simulink model "BATTERYLESS_SOLAR_INVERTER_DRIVE"  (R2021a)
settings: Solver=ode15s  StartTime=0.0  StopTime=inf  FixedStep=.00001  MaxStep=.00001  RelTol=1e-3  EnableMultiTasking=on
undefined symbols (not defined in the file): Capacitor, dEgdT, EgRef, gcbh, k1, Rsh_array5pc, Run, sps_rtmsupport, Start, Tref_K, VT_ref
libraries: fl_lib x7, spsCurrentMeasurementLib x6, nesl_utility x6, sh_lib x5, spsSeriesRLCBranchLib x5, spsIGBTDiodeLib x4, spsVoltageMeasurementLib x4, pid_lib x3, spsPVarrayModel x3, simulink x3, spsControlledCurrentSourceLib x2, spsRMSLib x2
(part 5 of 5)

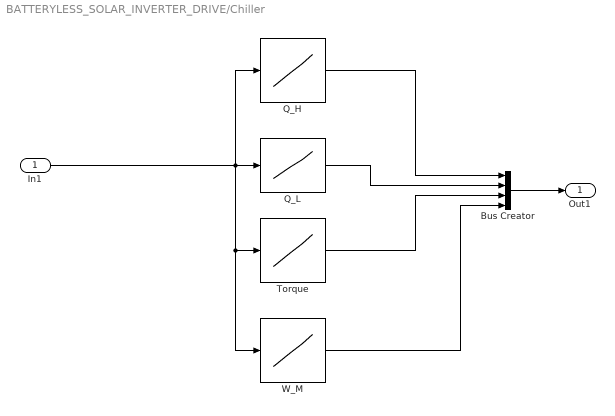
== system BATTERYLESS_SOLAR_INVERTER_DRIVE/Chiller ==
  In1 : Inport
  Bus Creator : BusCreator  Inputs=4
  Q_H : Lookup_n-D  NumberOfTableDimensions=1  BreakpointsForDimension1=|  Table=|  InternalRulePriority=Speed  RndMeth=Simplest  InputSameDT=on
      BreakpointsForDimension1=|
      | [0.16
      | 2.16
      | 4.16
      | 6.16
      | 8.16
      | 10.16
      | 12.16
      | 14.16
      | 16.16
      | 18.16
      | 20.16
      | 22.16
      | 24.16
      | 26.16
      | 28.16
      | 30.16
      | 32.16
      | 34.16
      | 36.16
      | 38.16
      | 40.16
      | 42.16
      | 44.16
      | 46.16
      | 48.16
      | 50.16
      | 52.16
      | 54.16
      | 56.16
      | 58.16
      | 60.16
      | 62.16
      | 64.16
      | 66.16
      | 68.16
      | 70.16
      | 72.16
      | 74.16
      | 76.16
      | 78.16
      | 80.16
      | 82.16
      | 84.16
      | 86.16
      | 88.16
      | 90.16
      | 92.16
      | 94.16
      | 96.16
      | 98.16
      | 100.2
      | 102.2
      | 104.2
      | 106.2
      | 108.2
      | 110.2
      | 112.2
      | 114.2
      | 116.2
      | 118.2
      | 120.2
      | 122.2
      | 124.2
      | 126.2
      | 128.2
      | 130.2
      | 132.2
      | 134.2
      | 136.2
      | 138.2
      | 140.2
      | 142.2
      | 144.2
      | 146.2
      | 148.2
      | 150.2
      | 152.2
      | 154.2
      | 156.2
      | 158.2
      | 160.2
      | 162.2
      | 164.2
      | 166.2
      | 168.2
      | 170.2
      | 172.2
      | 174.2
      | 176.2
      | 178.2
      | 180.2
      | 182.2
      | 184.2
      | 186.2
      | 188.2
      | 190.2
      | 192.2
      | 194.2
      | 196.2
      | 198.2
      | 200.2
      | 202.2
      | 204.2
      | 206.2
      | 208.2
      | 210.2
      | 212.2
      | 214.2
      | 216.2
      | 218.2
      | 220.2
      | 222.2
      | 224.2
      | 226.2
      | 228.2
      | 230.2
      | 232.2
      | 234.2
      | 236.2
      | 238.2
      | 240.2
      | 242.2
      | 244.2
      | 246.2
      | 248.2
      | 250.2
      | 252.2
      | 254.2
      | 256.2
      | 258.2
      | 260.2
      | 262.2
      | 264.2
      | 266.2
      | 268.2
      | 270.2
      | 272.2
      | 274.2
      | 276.2
      | 278.2
      | 280.2
      | 282.2
      | 284.2
      | 286.2
      | 288.2
      | 290.2
      | 292.2
      | 294.2
      | 296.2
      | 298.2
      | 300.2
      | 302.2
      | 304.2
      | 306.2
      | 308.2
      | 310.2
      | 312.2
      | 314.2
      | ]
      Table=|
      | [0.6508
      | 8.784
      | 16.92
      | 25.05
      | 33.18
      | 41.31
      | 49.43
      | 57.55
      | 65.67
      | 73.78
      | 81.88
      | 89.98
      | 98.07
      | 106.2
      | 114.2
      | 122.3
      | 130.4
      | 138.4
      | 146.4
      | 154.5
      | 162.5
      | 170.5
      | 178.5
      | 186.4
      | 194.4
      | 202.4
      | 210.3
      | 218.2
      | 226.1
      | 234
      | 241.9
      | 249.7
      | 257.6
      | 265.4
      | 273.2
      | 281
      | 288.8
      | 296.5
      | 304.2
      | 312
      | 319.6
      | 327.3
      | 335
      | 342.6
      | 350.2
      | 357.8
      | 365.4
      | 372.9
      | 380.4
      | 387.9
      | 395.4
      | 402.8
      | 410.3
      | 417.7
      | 425.1
      | 432.4
      | 439.8
      | 447.1
      | 454.4
      | 461.6
      | 468.9
      | 476.1
      | 483.3
      | 490.4
      | 497.6
      | 504.7
      | 511.8
      | 518.8
      | 525.9
      | 532.9
      | 539.9
      | 546.8
      | 553.8
      | 560.7
      | 567.5
      | 574.4
      | 581.2
      | 588
      | 594.8
      | 601.5
      | 608.2
      | 614.9
      | 621.6
      | 628.2
      | 634.8
      | 641.4
      | 647.9
      | 654.5
      | 661
      | 667.4
      | 673.9
      | 680.3
      | 686.6
      | 693
      | 699.3
      | 705.6
      | 711.9
      | 718.1
      | 724.3
      | 730.5
      | 736.6
      | 742.8
      | 748.8
      | 754.9
      | 760.9
      | 766.9
      | 772.9
      | 778.8
      | 784.7
      | 790.6
      | 796.5
      | 802.3
      | 808.1
      | 813.8
      | 819.6
      | 825.3
      | 830.9
      | 836.6
      | 842.2
      | 847.7
      | 853.3
      | 858.8
      | 864.3
      | 869.7
      | 875.1
      | 880.5
      | 885.9
      | 891.2
      | 896.5
      | 901.8
      | 907
      | 912.2
      | 917.4
      | 922.5
      | 927.6
      | 932.7
      | 937.7
      | 942.7
      | 947.7
      | 952.6
      | 957.5
      | 962.4
      | 967.3
      | 972.1
      | 976.8
      | 981.6
      | 986.3
      | 991
      | 995.6
      | 1000
      | 1005
      | 1009
      | 1014
      | 1018
      | 1023
      | 1027
      | 1032
      | 1036
      | ]
  Q_L : Lookup_n-D  NumberOfTableDimensions=1  BreakpointsForDimension1=|  Table=|  InternalRulePriority=Speed  RndMeth=Simplest  InputSameDT=on
      BreakpointsForDimension1=|
      | [0.16
      | 2.16
      | 4.16
      | 6.16
      | 8.16
      | 10.16
      | 12.16
      | 14.16
      | 16.16
      | 18.16
      | 20.16
      | 22.16
      | 24.16
      | 26.16
      | 28.16
      | 30.16
      | 32.16
      | 34.16
      | 36.16
      | 38.16
      | 40.16
      | 42.16
      | 44.16
      | 46.16
      | 48.16
      | 50.16
      | 52.16
      | 54.16
      | 56.16
      | 58.16
      | 60.16
      | 62.16
      | 64.16
      | 66.16
      | 68.16
      | 70.16
      | 72.16
      | 74.16
      | 76.16
      | 78.16
      | 80.16
      | 82.16
      | 84.16
      | 86.16
      | 88.16
      | 90.16
      | 92.16
      | 94.16
      | 96.16
      | 98.16
      | 100.2
      | 102.2
      | 104.2
      | 106.2
      | 108.2
      | 110.2
      | 112.2
      | 114.2
      | 116.2
      | 118.2
      | 120.2
      | 122.2
      | 124.2
      | 126.2
      | 128.2
      | 130.2
      | 132.2
      | 134.2
      | 136.2
      | 138.2
      | 140.2
      | 142.2
      | 144.2
      | 146.2
      | 148.2
      | 150.2
      | 152.2
      | 154.2
      | 156.2
      | 158.2
      | 160.2
      | 162.2
      | 164.2
      | 166.2
      | 168.2
      | 170.2
      | 172.2
      | 174.2
      | 176.2
      | 178.2
      | 180.2
      | 182.2
      | 184.2
      | 186.2
      | 188.2
      | 190.2
      | 192.2
      | 194.2
      | 196.2
      | 198.2
      | 200.2
      | 202.2
      | 204.2
      | 206.2
      | 208.2
      | 210.2
      | 212.2
      | 214.2
      | 216.2
      | 218.2
      | 220.2
      | 222.2
      | 224.2
      | 226.2
      | 228.2
      | 230.2
      | 232.2
      | 234.2
      | 236.2
      | 238.2
      | 240.2
      | 242.2
      | 244.2
      | 246.2
      | 248.2
      | 250.2
      | 252.2
      | 254.2
      | 256.2
      | 258.2
      | 260.2
      | 262.2
      | 264.2
      | 266.2
      | 268.2
      | 270.2
      | 272.2
      | 274.2
      | 276.2
      | 278.2
      | 280.2
      | 282.2
      | 284.2
      | 286.2
      | 288.2
      | 290.2
      | 292.2
      | 294.2
      | 296.2
      | 298.2
      | 300.2
      | 302.2
      | 304.2
      | 306.2
      | 308.2
      | 310.2
      | 312.2
      | 314.2
      | ]
      Table=|
      | [0.6507
      | 8.784
      | 16.92
      | 25.04
      | 33.17
      | 41.28
      | 49.38
      | 57.48
      | 65.56
      | 73.63
      | 81.68
      | 89.71
      | 97.72
      | 105.7
      | 113.7
      | 121.6
      | 129.5
      | 137.4
      | 145.3
      | 153.1
      | 160.9
      | 168.7
      | 176.4
      | 184.1
      | 191.8
      | 199.4
      | 207
      | 214.5
      | 222
      | 229.5
      | 236.9
      | 244.3
      | 251.6
      | 258.9
      | 266.2
      | 273.4
      | 280.5
      | 287.6
      | 294.7
      | 301.7
      | 308.7
      | 315.6
      | 322.5
      | 329.3
      | 336.1
      | 342.8
      | 349.5
      | 356.1
      | 362.6
      | 369.2
      | 375.6
      | 382
      | 388.4
      | 394.7
      | 401
      | 407.2
      | 413.4
      | 419.5
      | 425.5
      | 431.5
      | 437.5
      | 443.4
      | 449.2
      | 455
      | 460.8
      | 466.5
      | 472.1
      | 477.7
      | 483.2
      | 488.7
      | 494.2
      | 499.6
      | 504.9
      | 510.2
      | 515.4
      | 520.6
      | 525.7
      | 530.8
      | 535.8
      | 540.8
      | 545.7
      | 550.6
      | 555.5
      | 560.2
      | 565
      | 569.6
      | 574.3
      | 578.8
      | 583.4
      | 587.9
      | 592.3
      | 596.7
      | 601
      | 605.3
      | 609.5
      | 613.7
      | 617.8
      | 621.9
      | 626
      | 630
      | 633.9
      | 637.8
      | 641.6
      | 645.4
      | 649.2
      | 652.9
      | 656.5
      | 660.1
      | 663.7
      | 667.2
      | 670.7
      | 674.1
      | 677.4
      | 680.8
      | 684
      | 687.3
      | 690.4
      | 693.6
      | 696.7
      | 699.7
      | 702.7
      | 705.6
      | 708.5
      | 711.4
      | 714.2
      | 717
      | 719.7
      | 722.3
      | 724.9
      | 727.5
      | 730
      | 732.5
      | 735
      | 737.4
      | 739.7
      | 742
      | 744.2
      | 746.5
      | 748.6
      | 750.7
      | 752.8
      | 754.8
      | 756.8
      | 758.7
      | 760.6
      | 762.5
      | 764.3
      | 766
      | 767.7
      | 769.4
      | 771
      | 772.5
      | 774.1
      | 775.5
      | 777
      | 778.4
      | 779.7
      | 781
      | ]
  Torque : Lookup_n-D  NumberOfTableDimensions=1  BreakpointsForDimension1=|  Table=|  InternalRulePriority=Speed  RndMeth=Simplest  InputSameDT=on
      BreakpointsForDimension1=|
      | [0.16
      | 2.16
      | 4.16
      | 6.16
      | 8.16
      | 10.16
      | 12.16
      | 14.16
      | 16.16
      | 18.16
      | 20.16
      | 22.16
      | 24.16
      | 26.16
      | 28.16
      | 30.16
      | 32.16
      | 34.16
      | 36.16
      | 38.16
      | 40.16
      | 42.16
      | 44.16
      | 46.16
      | 48.16
      | 50.16
      | 52.16
      | 54.16
      | 56.16
      | 58.16
      | 60.16
      | 62.16
      | 64.16
      | 66.16
      | 68.16
      | 70.16
      | 72.16
      | 74.16
      | 76.16
      | 78.16
      | 80.16
      | 82.16
      | 84.16
      | 86.16
      | 88.16
      | 90.16
      | 92.16
      | 94.16
      | 96.16
      | 98.16
      | 100.2
      | 102.2
      | 104.2
      | 106.2
      | 108.2
      | 110.2
      | 112.2
      | 114.2
      | 116.2
      | 118.2
      | 120.2
      | 122.2
      | 124.2
      | 126.2
      | 128.2
      | 130.2
      | 132.2
      | 134.2
      | 136.2
      | 138.2
      | 140.2
      | 142.2
      | 144.2
      | 146.2
      | 148.2
      | 150.2
      | 152.2
      | 154.2
      | 156.2
      | 158.2
      | 160.2
      | 162.2
      | 164.2
      | 166.2
      | 168.2
      | 170.2
      | 172.2
      | 174.2
      | 176.2
      | 178.2
      | 180.2
      | 182.2
      | 184.2
      | 186.2
      | 188.2
      | 190.2
      | 192.2
      | 194.2
      | 196.2
      | 198.2
      | 200.2
      | 202.2
      | 204.2
      | 206.2
      | 208.2
      | 210.2
      | 212.2
      | 214.2
      | 216.2
      | 218.2
      | 220.2
      | 222.2
      | 224.2
      | 226.2
      | 228.2
      | 230.2
      | 232.2
      | 234.2
      | 236.2
      | 238.2
      | 240.2
      | 242.2
      | 244.2
      | 246.2
      | 248.2
      | 250.2
      | 252.2
      | 254.2
      | 256.2
      | 258.2
      | 260.2
      | 262.2
      | 264.2
      | 266.2
      | 268.2
      | 270.2
      | 272.2
      | 274.2
      | 276.2
      | 278.2
      | 280.2
      | 282.2
      | 284.2
      | 286.2
      | 288.2
      | 290.2
      | 292.2
      | 294.2
      | 296.2
      | 298.2
      | 300.2
      | 302.2
      | 304.2
      | 306.2
      | 308.2
      | 310.2
      | 312.2
      | 314.2
      | ]
      Table=|
      | [0.0001176
      | 0.0004362
      | 0.0007544
      | 0.0009557
      | 0.001676
      | 0.002595
      | 0.003712
      | 0.005025
      | 0.006533
      | 0.008233
      | 0.01012
      | 0.0122
      | 0.01446
      | 0.0169
      | 0.01952
      | 0.02232
      | 0.02528
      | 0.02842
      | 0.03171
      | 0.03517
      | 0.03878
      | 0.04253
      | 0.04644
      | 0.05049
      | 0.05467
      | 0.05899
      | 0.06344
      | 0.068
      | 0.07269
      | 0.0775
      | 0.08241
      | 0.08743
      | 0.09255
      | 0.09776
      | 0.1031
      | 0.1085
      | 0.1139
      | 0.1195
      | 0.1251
      | 0.1308
      | 0.1366
      | 0.1425
      | 0.1484
      | 0.1543
      | 0.1603
      | 0.1664
      | 0.1725
      | 0.1786
      | 0.1848
      | 0.191
      | 0.1973
      | 0.2036
      | 0.2099
      | 0.2163
      | 0.2226
      | 0.229
      | 0.2354
      | 0.2418
      | 0.2483
      | 0.2547
      | 0.2612
      | 0.2677
      | 0.2741
      | 0.2806
      | 0.2871
      | 0.2936
      | 0.3001
      | 0.3066
      | 0.313
      | 0.3195
      | 0.326
      | 0.3325
      | 0.3389
      | 0.3454
      | 0.3518
      | 0.3582
      | 0.3646
      | 0.371
      | 0.3774
      | 0.3838
      | 0.3902
      | 0.3965
      | 0.4028
      | 0.4091
      | 0.4154
      | 0.4217
      | 0.428
      | 0.4342
      | 0.4404
      | 0.4466
      | 0.4528
      | 0.4589
      | 0.4651
      | 0.4712
      | 0.4773
      | 0.4833
      | 0.4894
      | 0.4954
      | 0.5014
      | 0.5074
      | 0.5133
      | 0.5192
      | 0.5251
      | 0.531
      | 0.5368
      | 0.5427
      | 0.5485
      | 0.5542
      | 0.56
      | 0.5657
      | 0.5714
      | 0.5771
      | 0.5828
      | 0.5884
      | 0.594
      | 0.5996
      | 0.6051
      | 0.6106
      | 0.6161
      | 0.6216
      | 0.6271
      | 0.6325
      | 0.6379
      | 0.6432
      | 0.6486
      | 0.6539
      | 0.6592
      | 0.6645
      | 0.6697
      | 0.675
      | 0.6802
      | 0.6853
      | 0.6905
      | 0.6956
      | 0.7007
      | 0.7058
      | 0.7108
      | 0.7159
      | 0.7209
      | 0.7258
      | 0.7308
      | 0.7357
      | 0.7406
      | 0.7455
      | 0.7504
      | 0.7552
      | 0.76
      | 0.7648
      | 0.7696
      | 0.7743
      | 0.779
      | 0.7837
      | 0.7884
      | 0.793
      | 0.7977
      | 0.8023
      | 0.8069
      | 0.8114
      | ]
  W_M : Lookup_n-D  NumberOfTableDimensions=1  BreakpointsForDimension1=|  Table=|  InternalRulePriority=Speed  RndMeth=Simplest  InputSameDT=on
      BreakpointsForDimension1=|
      | [0.16
      | 2.16
      | 4.16
      | 6.16
      | 8.16
      | 10.16
      | 12.16
      | 14.16
      | 16.16
      | 18.16
      | 20.16
      | 22.16
      | 24.16
      | 26.16
      | 28.16
      | 30.16
      | 32.16
      | 34.16
      | 36.16
      | 38.16
      | 40.16
      | 42.16
      | 44.16
      | 46.16
      | 48.16
      | 50.16
      | 52.16
      | 54.16
      | 56.16
      | 58.16
      | 60.16
      | 62.16
      | 64.16
      | 66.16
      | 68.16
      | 70.16
      | 72.16
      | 74.16
      | 76.16
      | 78.16
      | 80.16
      | 82.16
      | 84.16
      | 86.16
      | 88.16
      | 90.16
      | 92.16
      | 94.16
      | 96.16
      | 98.16
      | 100.2
      | 102.2
      | 104.2
      | 106.2
      | 108.2
      | 110.2
      | 112.2
      | 114.2
      | 116.2
      | 118.2
      | 120.2
      | 122.2
      | 124.2
      | 126.2
      | 128.2
      | 130.2
      | 132.2
      | 134.2
      | 136.2
      | 138.2
      | 140.2
      | 142.2
      | 144.2
      | 146.2
      | 148.2
      | 150.2
      | 152.2
      | 154.2
      | 156.2
      | 158.2
      | 160.2
      | 162.2
      | 164.2
      | 166.2
      | 168.2
      | 170.2
      | 172.2
      | 174.2
      | 176.2
      | 178.2
      | 180.2
      | 182.2
      | 184.2
      | 186.2
      | 188.2
      | 190.2
      | 192.2
      | 194.2
      | 196.2
      | 198.2
      | 200.2
      | 202.2
      | 204.2
      | 206.2
      | 208.2
      | 210.2
      | 212.2
      | 214.2
      | 216.2
      | 218.2
      | 220.2
      | 222.2
      | 224.2
      | 226.2
      | 228.2
      | 230.2
      | 232.2
      | 234.2
      | 236.2
      | 238.2
      | 240.2
      | 242.2
      | 244.2
      | 246.2
      | 248.2
      | 250.2
      | 252.2
      | 254.2
      | 256.2
      | 258.2
      | 260.2
      | 262.2
      | 264.2
      | 266.2
      | 268.2
      | 270.2
      | 272.2
      | 274.2
      | 276.2
      | 278.2
      | 280.2
      | 282.2
      | 284.2
      | 286.2
      | 288.2
      | 290.2
      | 292.2
      | 294.2
      | 296.2
      | 298.2
      | 300.2
      | 302.2
      | 304.2
      | 306.2
      | 308.2
      | 310.2
      | 312.2
      | 314.2
      | ]
      Table=|
      | [0.0001724
      | 0.000363
      | 0.002592
      | 0.008411
      | 0.01953
      | 0.03766
      | 0.06448
      | 0.1017
      | 0.1508
      | 0.2136
      | 0.2915
      | 0.3862
      | 0.4991
      | 0.6317
      | 0.7854
      | 0.9616
      | 1.162
      | 1.387
      | 1.638
      | 1.917
      | 2.225
      | 2.562
      | 2.93
      | 3.329
      | 3.762
      | 4.227
      | 4.727
      | 5.262
      | 5.832
      | 6.439
      | 7.082
      | 7.763
      | 8.482
      | 9.24
      | 10.04
      | 10.87
      | 11.75
      | 12.66
      | 13.62
      | 14.61
      | 15.64
      | 16.72
      | 17.84
      | 18.99
      | 20.19
      | 21.43
      | 22.71
      | 24.03
      | 25.39
      | 26.79
      | 28.23
      | 29.71
      | 31.23
      | 32.8
      | 34.4
      | 36.04
      | 37.72
      | 39.44
      | 41.2
      | 43
      | 44.84
      | 46.71
      | 48.62
      | 50.58
      | 52.56
      | 54.59
      | 56.65
      | 58.75
      | 60.89
      | 63.06
      | 65.27
      | 67.52
      | 69.8
      | 72.11
      | 74.46
      | 76.84
      | 79.26
      | 81.71
      | 84.2
      | 86.72
      | 89.27
      | 91.85
      | 94.47
      | 97.12
      | 99.8
      | 102.5
      | 105.3
      | 108
      | 110.8
      | 113.7
      | 116.5
      | 119.4
      | 122.4
      | 125.3
      | 128.3
      | 131.3
      | 134.3
      | 137.4
      | 140.5
      | 143.6
      | 146.8
      | 150
      | 153.2
      | 156.4
      | 159.6
      | 162.9
      | 166.2
      | 169.6
      | 172.9
      | 176.3
      | 179.7
      | 183.2
      | 186.6
      | 190.1
      | 193.6
      | 197.1
      | 200.7
      | 204.3
      | 207.9
      | 211.5
      | 215.1
      | 218.8
      | 222.5
      | 226.2
      | 229.9
      | 233.7
      | 237.5
      | 241.3
      | 245.1
      | 248.9
      | 252.8
      | 256.7
      | 260.6
      | 264.5
      | 268.4
      | 272.4
      | 276.4
      | 280.4
      | 284.4
      | 288.4
      | 292.5
      | 296.6
      | 300.7
      | 304.8
      | 308.9
      | 313
      | 317.2
      | 321.4
      | 325.6
      | 329.8
      | 334
      | 338.3
      | 342.6
      | 346.9
      | 351.2
      | 355.5
      | 359.8
      | 364.2
      | ]
  Out1 : Outport
  wires:
  Q_H/1 -> Bus Creator/1
  Torque/1 -> Bus Creator/3
  In1/1 -> Q_H/1, W_M/1, Torque/1, Q_L/1
  Q_L/1 -> Bus Creator/2
  W_M/1 -> Bus Creator/4
  Bus Creator/1 -> Out1/1

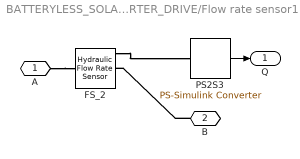
== system BATTERYLESS_SOLAR_INVERTER_DRIVE/Flow rate sensor1 ==
  FS_2 : fl_lib/Hydraulic/Hydraulic Sensors/Hydraulic Flow Rate Sensor  Tag=Factory Generic
  PS2S3 : nesl_utility/PS-Simulink Converter  PhysicalDomain=network_engine_domain  SubClassName=ps_output  LeftPortType=input  RightPortType=output  PseudoPeriodic=off  Frequencies=[]  Unit=1  AffineConversion=off
      settings: SourceProductBaseCode=PW,SS
  A : PMIOPort  Side=Left
  B : PMIOPort  Port=2  Side=Right
  Q : Outport  VectorParamsAs1DForOutWhenUnconnected=off
  wires:
  PS2S3/1 -> Q/1
  connections:
  B/RConn1 -- FS_2/RConn2
  A/RConn1 -- FS_2/LConn1
  FS_2/RConn1 -- PS2S3/LConn1

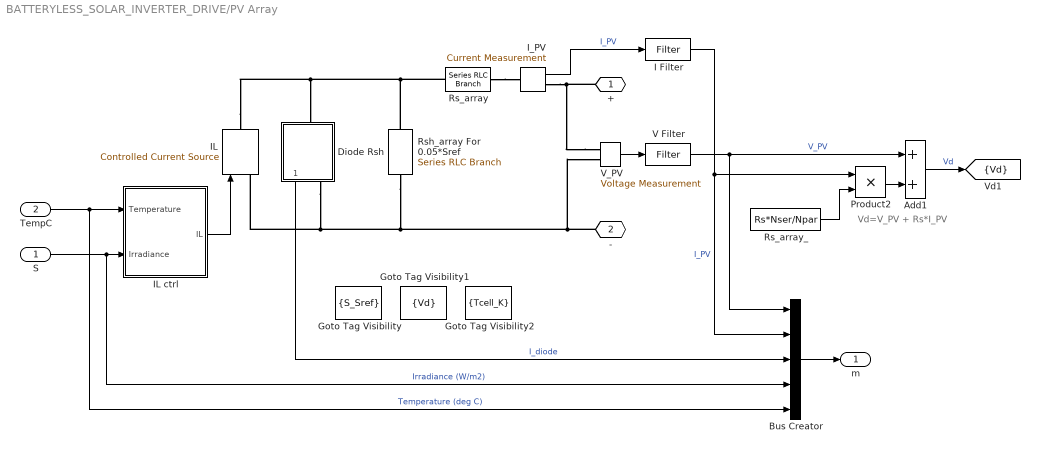
== system BATTERYLESS_SOLAR_INVERTER_DRIVE/PV Array ==
  note: Vd=V_PV + Rs*I_PV
  S : Inport
  TempC : Inport  Port=2
  Add1 : Sum
  Bus Creator : BusCreator  Inputs=5
  Diode Rsh : Subsystem
      mask Display:
      | plot(-75,-50,100,150, [-15 -15 43 -15 -15 -75],[50 8 50 92 50 50], ...
      |     [43 43],[8 94],[100 43], [50 50])
  Goto Tag Visibility : GotoTagVisibility  GotoTag=S_Sref
  Goto Tag Visibility1 : GotoTagVisibility  GotoTag=Vd
  Goto Tag Visibility2 : GotoTagVisibility  GotoTag=Tcell_K
  I Filter : spsPVarrayModel/Filter  SystemSampleTime=-1  VariantControl=Variant1  VariantActivationTime=update diagram  Latency=0  AutoFrameSizeCalculation=off
      settings: SourceProductBaseCode=PS
  IL : spsControlledCurrentSourceLib/Controlled Current Source  Initialize=on  Source_Type=AC  Amplitude=0  Phase=0  Frequency=0  Measurements=None
  IL ctrl : Subsystem
  I_PV : spsCurrentMeasurementLib/Current Measurement  PhasorSimulation=off  OutputType=Complex  PSBequivalent=0
  Product2 : Product  Inputs=**  RndMeth=Zero
  Rs_array : spsSeriesRLCBranchLib/Series RLC Branch  LConnTagsString=__new0  RConnTagsString=__new0  BranchType=R  Resistance=Rs*Nser/Npar  Inductance=1e-3  SetiL0=off  InitialCurrent=0  Capacitance=1e-6  Setx0=off  InitialVoltage=0  Measurements=None
  Rs_array_ : Constant  Value=Rs*Nser/Npar
  Rsh_array For 0.05*Sref : spsSeriesRLCBranchLib/Series RLC Branch  LConnTagsString=__new0  RConnTagsString=__new0  BranchType=R  Resistance=Rsh_array5pc  Inductance=1e-3  SetiL0=off  InitialCurrent=0  Capacitance=1e-6  Setx0=off  InitialVoltage=0  Measurements=None
  V Filter : spsPVarrayModel/Filter  SystemSampleTime=-1  VariantControl=Variant1  VariantActivationTime=update diagram  Latency=0  AutoFrameSizeCalculation=off
      settings: SourceProductBaseCode=PS
  V_PV : spsVoltageMeasurementLib/Voltage Measurement  PhasorSimulation=off  OutputType=Complex  PSBequivalent=0
  + : PMIOPort  Side=Right
  - : PMIOPort  Port=2  Side=Right
  m : Outport  VectorParamsAs1DForOutWhenUnconnected=off
  tag scope: Vd=scoped
  wires:
  V Filter/1 -> Add1/1, Bus Creator/1  "V_PV"
  I Filter/1 -> Product2/1, Bus Creator/2  "I_PV"
  V_PV/1 -> V Filter/1
  IL ctrl/1(IL) -> IL/1
  Bus Creator/1 -> m/1
  Rs_array_/1 -> Product2/2
  Product2/1 -> Add1/2
  I_PV/1 -> I Filter/1  "I_PV"
  Add1/1 -> [Vd]  "Vd"
  Diode Rsh/1(Idiode) -> Bus Creator/3  "I_diode"
  S/1 -> Bus Creator/4, IL ctrl/2(Irradiance)  "Irradiance (W/m2)"
  TempC/1 -> IL ctrl/1(Temperature), Bus Creator/5  "Temperature (deg C)"
  connections:
  Rs_array/RConn1 -- I_PV/LConn1
  IL/LConn1 -- Diode Rsh/RConn1 -- Rsh_array For 0.05*Sref/RConn1 -- -/RConn1 -- V_PV/LConn2
  IL/RConn1 -- Rsh_array For 0.05*Sref/LConn1 -- Rs_array/LConn1 -- Diode Rsh/LConn1
  V_PV/LConn1 -- I_PV/RConn1 -- +/RConn1

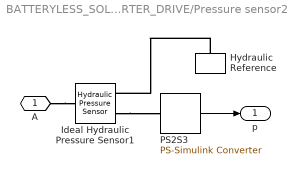
== system BATTERYLESS_SOLAR_INVERTER_DRIVE/Pressure sensor2 ==
  Hydraulic Reference : fl_lib/Hydraulic/Hydraulic Elements/Hydraulic Reference
  Ideal Hydraulic Pressure Sensor1 : fl_lib/Hydraulic/Hydraulic Sensors/Hydraulic Pressure Sensor  Tag=Factory Generic
  PS2S3 : nesl_utility/PS-Simulink Converter  PhysicalDomain=network_engine_domain  SubClassName=ps_output  LeftPortType=input  RightPortType=output  PseudoPeriodic=off  Frequencies=[]  Unit=bar  AffineConversion=off
      settings: SourceProductBaseCode=PW,SS
  A : PMIOPort  Side=Left
  p : Outport  VectorParamsAs1DForOutWhenUnconnected=off
  wires:
  PS2S3/1 -> p/1
  connections:
  A/RConn1 -- Ideal Hydraulic Pressure Sensor1/LConn1
  Hydraulic Reference/LConn1 -- Ideal Hydraulic Pressure Sensor1/RConn1
  Ideal Hydraulic Pressure Sensor1/RConn2 -- PS2S3/LConn1

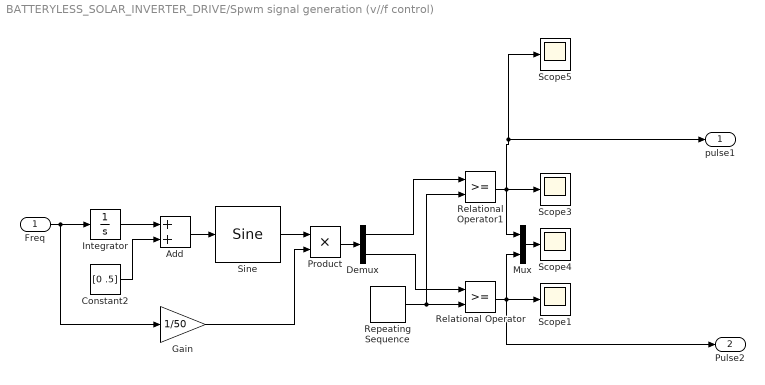
== system BATTERYLESS_SOLAR_INVERTER_DRIVE/Spwm signal generation (v//f control) ==
  Freq : Inport
  Add : Sum
  Constant2 : Constant  Value=[0 .5]
  Demux : Demux  Outputs=2
  Gain : Gain  Gain=1/50
  Integrator : Integrator
  Mux : Mux  Inputs=2
  Product : Product
  Relational Operator : RelationalOperator  OutDataTypeStr=boolean  RndMeth=Nearest
  Relational Operator1 : RelationalOperator  OutDataTypeStr=boolean  RndMeth=Nearest
  Repeating Sequence : simulink/Sources/Repeating Sequence  rep_seq_t=[0 .5 1]/8000  rep_seq_y=[0 1 0]
  Scope{1,3..5} (4 alike) : Scope
  Sine : simulink/Lookup Tables/Sine  Formula=sin(2*pi*u)  NumDataPoints=(2^5)+1  OutputWordLength=16  InternalRulePriority=Speed
  pulse1 : Outport  VectorParamsAs1DForOutWhenUnconnected=off
  Pulse2 : Outport  Port=2  VectorParamsAs1DForOutWhenUnconnected=off
  wires:
  Integrator/1 -> Add/1
  Demux/1 -> Relational Operator1/1
  Gain/1 -> Product/2
  Constant2/1 -> Add/2
  Product/1 -> Demux/1
  Add/1 -> Sine/1
  Repeating Sequence/1 -> Relational Operator1/2, Relational Operator/2
  Demux/2 -> Relational Operator/1
  Relational Operator/1 -> Pulse2/1, Mux/2, Scope1/1
  Mux/1 -> Scope4/1
  Sine/1 -> Product/1
  Relational Operator1/1 -> pulse1/1, Scope5/1, Mux/1, Scope3/1
  Freq/1 -> Gain/1, Integrator/1

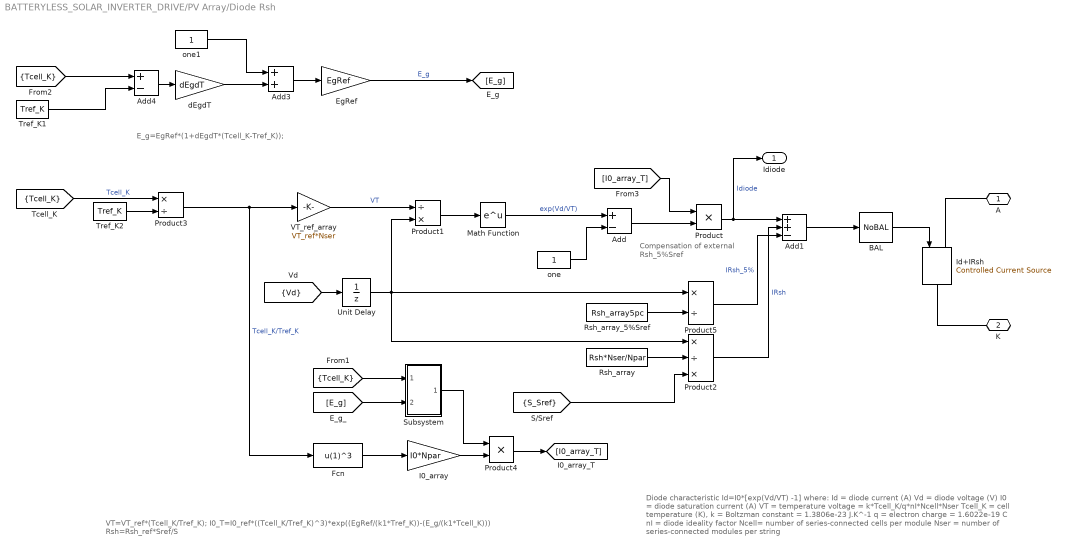
== system BATTERYLESS_SOLAR_INVERTER_DRIVE/PV Array/Diode Rsh ==
  note: Compensation of
      | external Rsh_5%Sref
  note: Diode characteristic
      |    Id=I0*[exp(Vd/VT) -1]
      |
      | where:
      |      Id = diode current (A)
      |      Vd = diode voltage (V)
      |      I0 = diode saturation current (A)
      |      VT = temperature voltage = k*Tcell_K/q*nI*Ncell*Nser
      | Tcell_K = cell temperature (K),
      |       k = Boltzman constant = 1.3806e-23 J.K^-1
      |       q = electron charge = 1.6022e-19 C
      |      nI = diode ideality factor
      |    Ncell= number of series-connected cells per module
      |    Nser = number of series-connected modules per string
  note: VT=VT_ref*(Tcell_K/Tref_K);
      | I0_T=I0_ref*((Tcell_K/Tref_K)^3)*exp((EgRef/(k1*Tref_K))-(E_g/(k1*Tcell_K)))
      | Rsh=Rsh_ref*Sref/S
  note: E_g=EgRef*(1+dEgdT*(Tcell_K-Tref_K));
  Add : Sum  Inputs=+-
  Add1 : Sum  Inputs=++-
  Add3 : Sum
  Add4 : Sum  Inputs=+-
  BAL : spsPVarrayModel/NoBAL  SystemSampleTime=-1  VariantControl=NoBAL
      settings: SourceProductBaseCode=PS
  EgRef : Gain  Gain=EgRef
  Fcn : Fcn  Expr=u(1)^3
  I0_array : Gain  Gain=I0*Npar
  Id+IRsh : spsControlledCurrentSourceLib/Controlled Current Source  Initialize=on  Source_Type=AC  Amplitude=0  Phase=0  Frequency=0  Measurements=None
  Math Function : Math  SignedPower=on  SaturateOnIntegerOverflow=on
  Product : Product  RndMeth=Zero
  Product1 : Product  Inputs=/*  RndMeth=Zero
  Product2 : Product  Inputs=*/*  RndMeth=Zero
  Product3 : Product  Inputs=*/  RndMeth=Zero
  Product4 : Product  Inputs=**  RndMeth=Zero
  Product5 : Product  Inputs=*/  RndMeth=Zero
  Rsh_array : Constant  Value=Rsh*Nser/Npar
  Rsh_array_5%Sref : Constant  Value=Rsh_array5pc
  Subsystem : Subsystem
  Tref_K1 : Constant  Value=Tref_K
  Tref_K2 : Constant  Value=Tref_K
  Unit Delay : UnitDelay  SampleTime=-1  HasFrameUpgradeWarning=on
  VT_ref_array : Gain  Gain=VT_ref*Nser
  dEgdT : Gain  Gain=dEgdT
  one : Constant
  one1 : Constant
  A : PMIOPort  Side=Left
  K : PMIOPort  Port=2  Side=Right
  Idiode : Outport  VectorParamsAs1DForOutWhenUnconnected=off
  wires:
  BAL/1 -> Id+IRsh/1
  Add1/1 -> BAL/1
  Product5/1 -> Add1/3  "IRsh_5%"
  Rsh_array_5%Sref/1 -> Product5/2
  Math Function/1 -> Add/1  "exp(Vd/VT)"
  Product2/1 -> Add1/2  "IRsh"
  Product/1 -> Add1/1, Idiode/1  "Idiode"
  Product1/1 -> Math Function/1
  one/1 -> Add/2
  Rsh_array/1 -> Product2/2
  [Tcell_K] -> Product3/1  "Tcell_K"
  Product3/1 -> VT_ref_array/1, Fcn/1  "Tcell_K/Tref_K"
  one1/1 -> Add3/1
  Add4/1 -> dEgdT/1
  dEgdT/1 -> Add3/2
  Add3/1 -> EgRef/1
  EgRef/1 -> [E_g]  "E_g"
  I0_array/1 -> Product4/2
  Fcn/1 -> I0_array/1
  [Tcell_K] -> Add4/1
  Tref_K1/1 -> Add4/2
  Subsystem/1(exp) -> Product4/1
  [Tcell_K] -> Subsystem/1(Tcell_K)
  [E_g] -> Subsystem/2(E_g)
  Tref_K2/1 -> Product3/2
  Product4/1 -> [I0_array_T]
  Add/1 -> Product/2
  VT_ref_array/1 -> Product1/1  "VT"
  [I0_array_T] -> Product/1
  [Vd] -> Unit Delay/1
  [S_Sref] -> Product2/3
  Unit Delay/1 -> Product5/1, Product2/1, Product1/2
  connections:
  Id+IRsh/RConn1 -- K/RConn1
  A/RConn1 -- Id+IRsh/LConn1

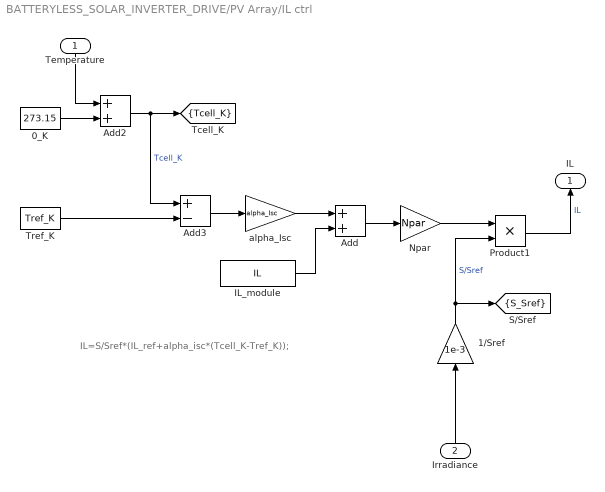
== system BATTERYLESS_SOLAR_INVERTER_DRIVE/PV Array/IL ctrl ==
  note: IL=S/Sref*(IL_ref+alpha_isc*(Tcell_K-Tref_K));
  Temperature : Inport
  Irradiance : Inport  Port=2
  0_K : Constant  Value=273.15
  1/Sref : Gain  Gain=1e-3
  Add : Sum
  Add2 : Sum
  Add3 : Sum  Inputs=+-
  IL_module : Constant  Value=IL
  Npar : Gain  Gain=Npar
  Product1 : Product  Inputs=**  RndMeth=Zero
  Tref_K : Constant  Value=Tref_K
  alpha_Isc : Gain  Gain=alpha_Isc
  IL : Outport  VectorParamsAs1DForOutWhenUnconnected=off
  tag scope: S_Sref=scoped, Tcell_K=scoped
  wires:
  Temperature/1 -> Add2/1
  Irradiance/1 -> 1/Sref/1
  alpha_Isc/1 -> Add/1
  Add3/1 -> alpha_Isc/1
  Tref_K/1 -> Add3/2
  Product1/1 -> IL/1  "IL"
  IL_module/1 -> Add/2
  0_K/1 -> Add2/2
  Add/1 -> Npar/1
  Add2/1 -> Add3/1, [Tcell_K]  "Tcell_K"
  Npar/1 -> Product1/1
  1/Sref/1 -> Product1/2, [S_Sref]  "S/Sref"

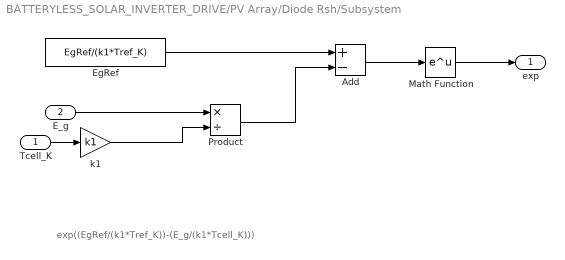
== system BATTERYLESS_SOLAR_INVERTER_DRIVE/PV Array/Diode Rsh/Subsystem ==
  note: exp((EgRef/(k1*Tref_K))-(E_g/(k1*Tcell_K)))
  Tcell_K : Inport
  E_g : Inport  Port=2
  Add : Sum  Inputs=+-
  EgRef : Constant  Value=EgRef/(k1*Tref_K)
  Math Function : Math  SignedPower=on  SaturateOnIntegerOverflow=on
  Product : Product  Inputs=*/
  k1 : Gain  Gain=k1
  exp : Outport  VectorParamsAs1DForOutWhenUnconnected=off
  wires:
  EgRef/1 -> Add/1
  E_g/1 -> Product/1
  Tcell_K/1 -> k1/1
  k1/1 -> Product/2
  Product/1 -> Add/2
  Add/1 -> Math Function/1
  Math Function/1 -> exp/1

== stateflow chart BATTERYLESS_SOLAR_INVERTER_DRIVE/Inc Cond Method1 ==
  settings: updateMethod=DISCRETE  sampleTime=1e-4
  state SAMPLEandCALCULATE
    entry:
    deltaV = Vpv - Vprev;
    deltaI = Ipv - Iprev;
    d = D;
  state INCREMENT_DUTY
    entry:
    d = d + deltad;
  state DECREMENT_DUTY
    entry:
    d = d - deltad;
  state RETURN
    entry:
    Vprev = Vpv; Iprev = Ipv;
    D = d;
  RETURN -> SAMPLEandCALCULATE
  (default) -> SAMPLEandCALCULATE
  SAMPLEandCALCULATE -> (junction 14) [order 1] : [deltaV > Vtol || deltaV < -Vtol]
  SAMPLEandCALCULATE -> (junction 15) [order 2]
  (junction 15) -> RETURN [order 3]
  (junction 15) -> INCREMENT_DUTY [order 1] : [deltaI < -Itol]
  (junction 14) -> RETURN [order 3]
  (junction 14) -> DECREMENT_DUTY [order 1] : [deltaI/deltaV > -Ipv/Vpv]
  (junction 14) -> INCREMENT_DUTY [order 2] : [deltaI/deltaV < -Ipv/Vpv]
  (junction 15) -> DECREMENT_DUTY [order 2] : [deltaI > Itol]
  INCREMENT_DUTY -> RETURN
  DECREMENT_DUTY -> RETURN
  data: Vpv input; Ipv input; D output double =0.67; Vprev local double =0; Iprev local double =0; Itol constant double =0.001; Vtol constant double =0.001; deltad constant double =0.0025; deltaV local double =0; deltaI local double =0; d local double =0
